simulink model "chap2_7sim"  (Simulink 8.1)
settings: Solver=ode5  StartTime=0.0  StopTime=3  FixedStep=0.001  RelTol=1e-3
settings Model: Creator=ljk  LastModifiedBy=liujk  ExtModeTrigMode=oneshot  ExtModeArmWhenConnect=off
settings DataIOCC: LimitDataPoints=off  SignalLoggingName=sigsOut
settings OptimizationCC: BooleanDataType=off
settings DebuggingCC: SaveWithParameterizedLinksMsg=none  SignalResolutionControl=TryResolveAllWithWarning  SolverPrmCheckMsg=none  MultiTaskDSMMsg=warning  MultiTaskCondExecSysMsg=none  StrictBusMsg=None
settings HardwareCC: TargetUnknown=on
settings RTWCC: IncludeERTFirstTime=on

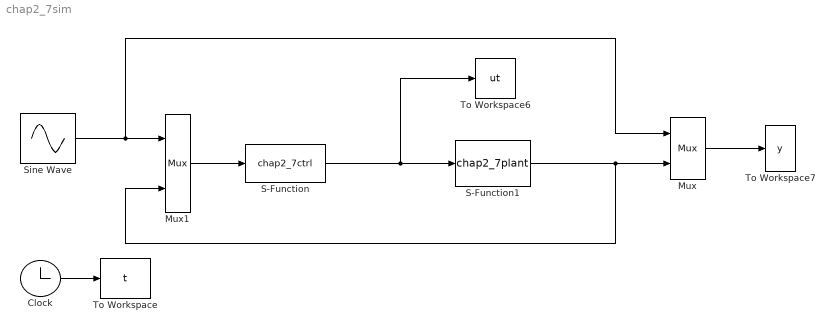
== system chap2_7sim ==
  Clock : Clock
  Mux : Mux  Inputs=2
  Mux1 : Mux  Inputs=2
  S-Function : S-Function  FunctionName=chap2_7ctrl  EnableBusSupport=off
  S-Function1 : S-Function  FunctionName=chap2_7plant  EnableBusSupport=off
  Sine Wave : Sin  Frequency=2*pi  SampleTime=0
  To Workspace : ToWorkspace  VariableName=t  SampleTime=-1
  To Workspace6 : ToWorkspace  VariableName=ut  SampleTime=-1
  To Workspace7 : ToWorkspace  VariableName=y  SampleTime=-1
  wires:
  Clock/1 -> To Workspace/1
  S-Function1/1 -> Mux1/2, Mux/2
  Mux/1 -> To Workspace7/1
  Mux1/1 -> S-Function/1
  Sine Wave/1 -> Mux/1, Mux1/1
  S-Function/1 -> To Workspace6/1, S-Function1/1
